simulink model "Step_response_SS_PID"  (R2017b)
settings: Solver=VariableStepAuto  StartTime=0.0  StopTime=10.0  RelTol=1e-3
values from neighbouring files (symbols this model uses):
  g = 9.81    [RWIP_2axis.m]
  Ip = 8.049E-3    (= 0.008049)    [RWIP_2axis.m]
  Iw = 8.06E-5    (= 8.06e-05)    [RWIP_2axis.m]
  Km = 3.7E-2    (= 0.037)    [RWIP_2axis.m]
  lp = 0.331    [RWIP_2axis.m]
  lw = 0.369    [RWIP_2axis.m]
  mp = 0.533    [RWIP_2axis.m]
  mw = 0.107    [RWIP_2axis.m]
  x0 = [pi/30;0;0]    [RWIP_2axis.m]
settings Model: Creator=Utilisateur  LastModifiedBy=Utilisateur

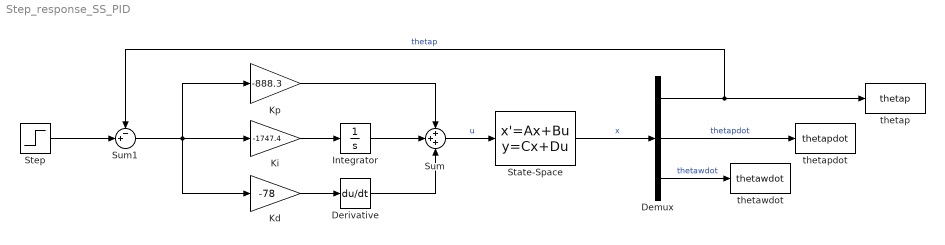
== system Step_response_SS_PID ==
  Demux : Demux  Outputs=3
  Derivative : Derivative
  Integrator : Integrator
  Kd : Gain  Gain=-78
  Ki : Gain  Gain=-1747.4
  Kp : Gain  Gain=-888.3
  State-Space : StateSpace  A=[0 1 0;(mp*lp+mw*lw)*g/(mp*lp^2+mw*lw^2+Ip) 0 0;(mp*lp+mw*lw)*g/(-(mp*lp^2+mw*lw^2+Ip)) 0 0]  B=[0; -Km/(mp*lp^2+mw*lw^2+Ip); Km*(mp*lp^2+mw*lw^2+Ip+Iw)/(Iw*(mp*lp^2+mw*lw^2+Ip))]  C=eye(3)  D=[0; 0; 0]  InitialCondition=x0  ContinuousStateAttributes={'thetap', 'thetapdot', 'thetawdot'}
  Step : Step  Time=0  SampleTime=0
  Sum : Sum  Inputs=+++
  Sum1 : Sum  Inputs=-+|
  thetap : ToWorkspace  VariableName=thetap  SaveFormat=Structure With Time  SampleTime=-1
  thetapdot : ToWorkspace  VariableName=thetapdot  SaveFormat=Structure With Time  SampleTime=-1
  thetawdot : ToWorkspace  VariableName=thetawdot  SaveFormat=Structure With Time  SampleTime=-1
  wires:
  Demux/1 -> thetap/1, Sum1/1  "thetap"
  State-Space/1 -> Demux/1  "x"
  Demux/3 -> thetawdot/1  "thetawdot"
  Demux/2 -> thetapdot/1  "thetapdot"
  Kd/1 -> Derivative/1
  Sum/1 -> State-Space/1  "u"
  Kp/1 -> Sum/1
  Step/1 -> Sum1/2
  Sum1/1 -> Ki/1, Kp/1, Kd/1
  Derivative/1 -> Sum/3
  Ki/1 -> Integrator/1
  Integrator/1 -> Sum/2
